simulink model "DP"  (Simulink 7.3)
settings: Solver=ode5  StartTime=0.0  StopTime=inf  FixedStep=0.1  RelTol=1e-3
undefined symbols (not defined in the file): eta1_0_real, v1_0_real, velocitySatValues1
libraries: simulink x18, marine_gnc x4, dspinverses x1, simulink_extras x1
(part 1 of 2)
settings Model: Creator=Dinh  LastModifiedBy=mcl  BufferReuse=off
settings DataIOCC: LimitDataPoints=off  SaveOutput=off  SaveTime=off
settings OptimizationCC: BlockReduction=off  BooleanDataType=off  ConditionallyExecuteInputs=off  OptimizeBlockIOStorage=off  BufferReuse=off  ExpressionFolding=off  LocalBlockOutputs=off  SimCompilerOptimization=On
settings SFSimCC: SimBuildMode=sf_nonincremental_build
settings RTWCC: SystemTargetFile=nidll_vxworks.tlc  TemplateMakefile=nidll_vxworks.tmf  Description=NI Real-Time VxWorks Target for Release 2007b or later  ProcessScript=nidll_vxworks_make_rtw_hook  RTWCompilerOptimization=On
settings STFCustomTargetCC: MatFileLogging=on  SystemTargetFile=nidll_vxworks.tlc

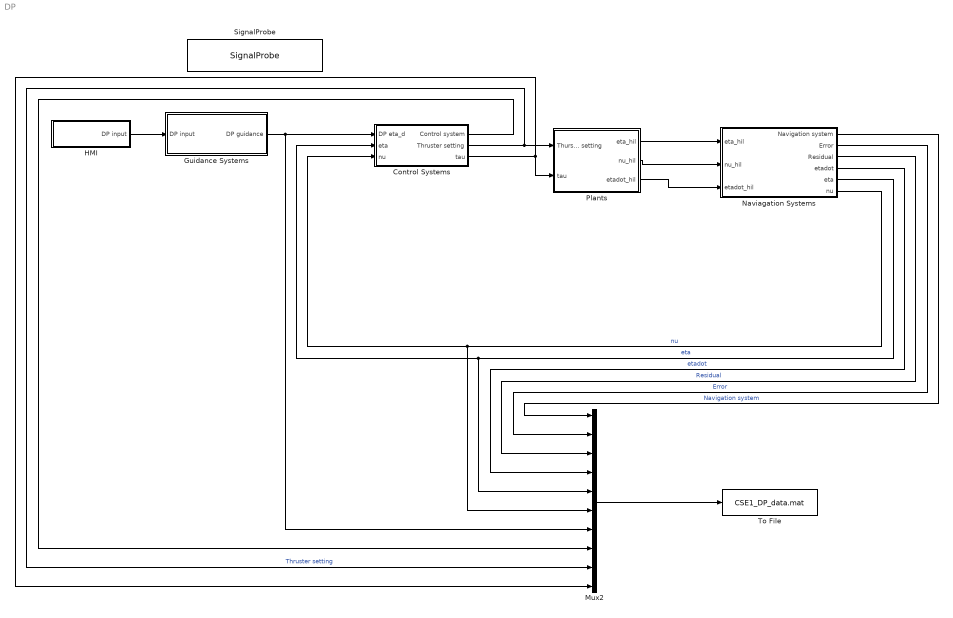
== system DP ==
  Control Systems : Subsystem
  Guidance Systems : Subsystem
  HMI : Subsystem
  Mux2 : Mux  Inputs=10
  Naviagation Systems : Subsystem
      settings: MinAlgLoopOccurrences=on
  Plants : Subsystem
  SignalProbe : S-Function  Description=Use this block with SIT.  FunctionName=SignalProbe  Parameters=1  EnableBusSupport=off
      settings: PreSaveFcn=NISIT_ModelVars;
      mask Description: The LabVIEW Simulation Interface Toolkit uses the SignalProbe block to probe the signals in the model. The SignalProbe block must be on the top level of the model hierarchy. You can have only one SignalProbe block per model file. Do not rename the SignalProbe block. Do not change the name of another model block to SignalProbe.
  To File : ToFile  Filename=CSE1_DP_data.mat  MatrixName=cse1_DP_data
  wires:
  HMI/1(DP input) -> Guidance Systems/1(DP input)
  Guidance Systems/1(DP guidance) -> Control Systems/1(DP eta_d), Mux2/7
  Plants/1(eta_hil) -> Naviagation Systems/1(eta_hil)
  Plants/2(nu_hil) -> Naviagation Systems/2(nu_hil)
  Plants/3(etadot_hil) -> Naviagation Systems/3(etadot_hil)
  Naviagation Systems/5(eta) -> Control Systems/2(eta), Mux2/5  "eta"
  Naviagation Systems/6(nu) -> Mux2/6, Control Systems/3(nu)  "nu"
  Naviagation Systems/3(Residual) -> Mux2/3  "Residual"
  Naviagation Systems/4(etadot) -> Mux2/4  "etadot"
  Naviagation Systems/2(Error) -> Mux2/2  "Error"
  Naviagation Systems/1(Navigation system) -> Mux2/1  "Navigation system"
  Mux2/1 -> To File/1
  Control Systems/1(Control system) -> Mux2/8
  Control Systems/3(tau) -> Mux2/10, Plants/2(tau)
  Control Systems/2(Thruster setting) -> Mux2/9, Plants/1(Thurster setting)  "Thruster setting"

== system DP/Control Systems ==
  note: 0 - PS3 u input control
      | 1 - DP control
  DP eta_d : Inport
  eta : Inport  Port=2
  nu : Inport  Port=3
  Control Mode : Constant  Value=0
  DP control : Subsystem
  PS3 input : Subsystem
  PS3 u input control : Subsystem
      settings: MinAlgLoopOccurrences=on
  Saturation : Saturate  UpperLimit=1.0  LowerLimit=-1.0
  Thruster setting Switch : MultiPortSwitch  Inputs=2  zeroidx=on
  tau Switch : MultiPortSwitch  Inputs=2  zeroidx=on
  Control system : Outport
  Thruster setting : Outport  Port=2
  tau : Outport  Port=3
  wires:
  Thruster setting Switch/1 -> Saturation/1
  Saturation/1 -> Thruster setting/1
  Control Mode/1 -> Thruster setting Switch/1, Control system/1, tau Switch/1
  PS3 u input control/1(Thruster setting) -> Thruster setting Switch/2
  PS3 input/1(DuelShock 3 signals) -> PS3 u input control/1(PS3 Signals)
  PS3 input/2(PS3 BT Power) -> PS3 u input control/2(PS3 BT Power)
  PS3 input/3(PS3 VSP Speed) -> PS3 u input control/3(PS3 VSP Speed)
  DP eta_d/1 -> DP control/1(eta_d)
  eta/1 -> DP control/2(eta)
  nu/1 -> DP control/3(nu)
  DP control/1(Thruster setting) -> Thruster setting Switch/3
  tau Switch/1 -> tau/1
  PS3 u input control/2(tau) -> tau Switch/2
  DP control/2(tau) -> tau Switch/3

== system DP/Guidance Systems ==
  DP input : Inport
  DP : Subsystem
  DP guidance : Outport
  wires:
  DP/1(DP eta_d) -> DP guidance/1
  DP input/1 -> DP/1(DP input)

== system DP/HMI ==
  Battery Bow Thruster : Gain  ParameterDataType=fixdt(1, 16)  ParameterScaling=2^0  OutDataType=fixdt(1, 16)  OutScaling=2^0
  Battery Main : Gain  Gain=2  ParameterDataType=fixdt(1, 16)  ParameterScaling=2^0  OutDataType=fixdt(1, 16)  OutScaling=2^0
  Battery Servo : Gain  ParameterDataType=fixdt(1, 16)  ParameterScaling=2^0  OutDataType=fixdt(1, 16)  OutScaling=2^0
  DP Input : Subsystem
  SIT zAI0 : S-Function  Priority=1  FunctionName=NI_SIT_IO  Parameters=width dtype portnum stime stype btype  EnableBusSupport=off  mask(SIT Inport){portnum=1, width=-1, stime=-1, dtype=auto, stype=auto, btype=1}
      mask prompts: portnum "Port number:"; width "Port dimensions (-1 for dynamically sized):"; stime "Sample time (-1 for inherited):"; dtype "Data type:"; stype "Signal type:"; btype "Block type:"
      mask help: Use this inport on any level of nested subsystems to allow the LabVIEW Simulation Interface Toolkit to map hardware to it.
      mask init:
      | NI_SIT_IO_init;
      settings: CopyFcn=NI_SIT_IO_callbacks(1);  DeleteFcn=NI_SIT_IO_callbacks(2);
      mask StyleString: edit,edit,edit,popup(auto|double|single|int8|uint8|int16|uint16|int32|uint32|boolean),popup(auto|real|complex),edit
      mask CallbackString: NI_SIT_IO_callbacks(3);|||NI_SIT_IO_callbacks(4);||
      mask TabNameString: Parameters,Parameters,Parameters,Parameters,Parameters,Parameters
      mask Display:
      | patch([-x x], [-y y], [.90980 .81960 .32156]);
      | plot([0 -x x 0], [rad -y y rad]);
      | fprintf('SIT%d', portnum);
  SIT zAI1 : S-Function  Priority=2  FunctionName=NI_SIT_IO  Parameters=width dtype portnum stime stype btype  EnableBusSupport=off  mask(SIT Inport){portnum=2, width=-1, stime=-1, dtype=auto, stype=auto, btype=1}
      mask prompts: portnum "Port number:"; width "Port dimensions (-1 for dynamically sized):"; stime "Sample time (-1 for inherited):"; dtype "Data type:"; stype "Signal type:"; btype "Block type:"
      mask help: Use this inport on any level of nested subsystems to allow the LabVIEW Simulation Interface Toolkit to map hardware to it.
      mask init:
      | NI_SIT_IO_init;
      settings: CopyFcn=NI_SIT_IO_callbacks(1);  DeleteFcn=NI_SIT_IO_callbacks(2);
      mask StyleString: edit,edit,edit,popup(auto|double|single|int8|uint8|int16|uint16|int32|uint32|boolean),popup(auto|real|complex),edit
      mask CallbackString: NI_SIT_IO_callbacks(3);|||NI_SIT_IO_callbacks(4);||
      mask TabNameString: Parameters,Parameters,Parameters,Parameters,Parameters,Parameters
      mask Display:
      | patch([-x x], [-y y], [.90980 .81960 .32156]);
      | plot([0 -x x 0], [rad -y y rad]);
      | fprintf('SIT%d', portnum);
  SIT zAI2 : S-Function  Priority=3  FunctionName=NI_SIT_IO  Parameters=width dtype portnum stime stype btype  EnableBusSupport=off  mask(SIT Inport){portnum=3, width=-1, stime=-1, dtype=auto, stype=auto, btype=1}
      mask prompts: portnum "Port number:"; width "Port dimensions (-1 for dynamically sized):"; stime "Sample time (-1 for inherited):"; dtype "Data type:"; stype "Signal type:"; btype "Block type:"
      mask help: Use this inport on any level of nested subsystems to allow the LabVIEW Simulation Interface Toolkit to map hardware to it.
      mask init:
      | NI_SIT_IO_init;
      settings: CopyFcn=NI_SIT_IO_callbacks(1);  DeleteFcn=NI_SIT_IO_callbacks(2);
      mask StyleString: edit,edit,edit,popup(auto|double|single|int8|uint8|int16|uint16|int32|uint32|boolean),popup(auto|real|complex),edit
      mask CallbackString: NI_SIT_IO_callbacks(3);|||NI_SIT_IO_callbacks(4);||
      mask TabNameString: Parameters,Parameters,Parameters,Parameters,Parameters,Parameters
      mask Display:
      | patch([-x x], [-y y], [.90980 .81960 .32156]);
      | plot([0 -x x 0], [rad -y y rad]);
      | fprintf('SIT%d', portnum);
  Terminator Bow Thruster Battery : Terminator
  Terminator Main Battery : Terminator
  Terminator Servo Battery : Terminator
  DP input : Outport
  wires:
  SIT zAI0/1 -> Battery Bow Thruster/1
  SIT zAI1/1 -> Battery Servo/1
  SIT zAI2/1 -> Battery Main/1
  Battery Bow Thruster/1 -> Terminator Bow Thruster Battery/1
  Battery Servo/1 -> Terminator Servo Battery/1
  Battery Main/1 -> Terminator Main Battery/1
  DP Input/1(DP input) -> DP input/1

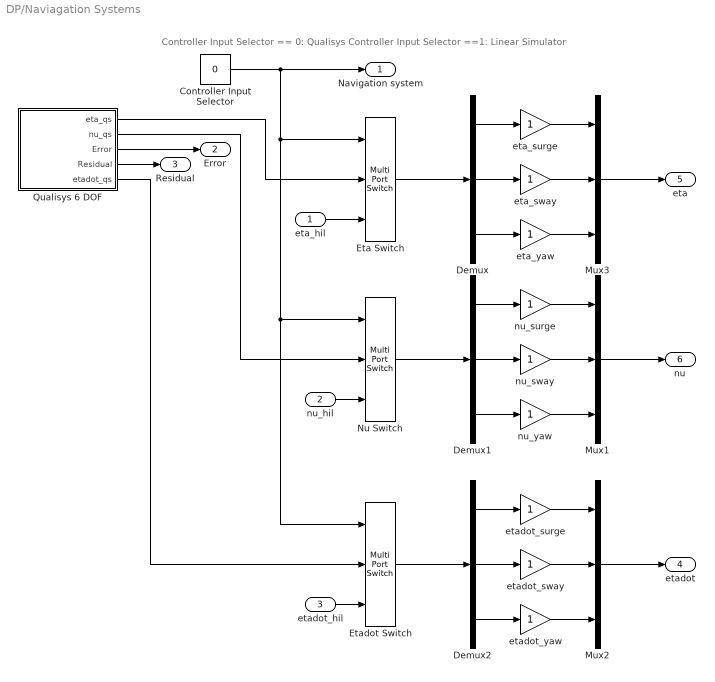
== system DP/Naviagation Systems ==
  note: Controller Input Selector == 0: Qualisys
      | Controller Input Selector ==1: Linear Simulator
  eta_hil : Inport
  nu_hil : Inport  Port=2
  etadot_hil : Inport  Port=3
  Controller Input Selector : Constant  Value=0
  Demux : Demux  Outputs=3
  Demux1 : Demux  Outputs=3
  Demux2 : Demux  Outputs=3
  Eta Switch : MultiPortSwitch  Inputs=2  zeroidx=on
  Etadot Switch : MultiPortSwitch  Inputs=2  zeroidx=on
  Mux1 : Mux  Inputs=3
  Mux2 : Mux  Inputs=3
  Mux3 : Mux  Inputs=3
  Nu Switch : MultiPortSwitch  Inputs=2  zeroidx=on
  Qualisys 6 DOF : Subsystem
  eta_surge : Gain  ParameterDataType=fixdt(1, 16)  ParameterScaling=2^0  OutDataType=fixdt(1, 16)  OutScaling=2^0
  eta_sway : Gain  ParameterDataType=fixdt(1, 16)  ParameterScaling=2^0  OutDataType=fixdt(1, 16)  OutScaling=2^0
  eta_yaw : Gain  ParameterDataType=fixdt(1, 16)  ParameterScaling=2^0  OutDataType=fixdt(1, 16)  OutScaling=2^0
  etadot_surge : Gain  ParameterDataType=fixdt(1, 16)  ParameterScaling=2^0  OutDataType=fixdt(1, 16)  OutScaling=2^0
  etadot_sway : Gain  ParameterDataType=fixdt(1, 16)  ParameterScaling=2^0  OutDataType=fixdt(1, 16)  OutScaling=2^0
  etadot_yaw : Gain  ParameterDataType=fixdt(1, 16)  ParameterScaling=2^0  OutDataType=fixdt(1, 16)  OutScaling=2^0
  nu_surge : Gain  ParameterDataType=fixdt(1, 16)  ParameterScaling=2^0  OutDataType=fixdt(1, 16)  OutScaling=2^0
  nu_sway : Gain  ParameterDataType=fixdt(1, 16)  ParameterScaling=2^0  OutDataType=fixdt(1, 16)  OutScaling=2^0
  nu_yaw : Gain  ParameterDataType=fixdt(1, 16)  ParameterScaling=2^0  OutDataType=fixdt(1, 16)  OutScaling=2^0
  Navigation system : Outport
  Error : Outport  Port=2
  Residual : Outport  Port=3
  etadot : Outport  Port=4
  eta : Outport  Port=5
  nu : Outport  Port=6
  wires:
  Controller Input Selector/1 -> Eta Switch/1, Nu Switch/1, Etadot Switch/1, Navigation system/1
  Qualisys 6 DOF/1(eta_qs) -> Eta Switch/2
  Qualisys 6 DOF/2(nu_qs) -> Nu Switch/2
  eta_hil/1 -> Eta Switch/3
  nu_hil/1 -> Nu Switch/3
  Demux/1 -> eta_surge/1
  Demux/2 -> eta_sway/1
  Demux/3 -> eta_yaw/1
  eta_surge/1 -> Mux3/1
  eta_yaw/1 -> Mux3/3
  eta_sway/1 -> Mux3/2
  Mux3/1 -> eta/1
  Demux1/1 -> nu_surge/1
  Demux1/2 -> nu_sway/1
  Demux1/3 -> nu_yaw/1
  nu_surge/1 -> Mux1/1
  nu_sway/1 -> Mux1/2
  nu_yaw/1 -> Mux1/3
  Mux1/1 -> nu/1
  Nu Switch/1 -> Demux1/1
  Eta Switch/1 -> Demux/1
  Qualisys 6 DOF/3(Error) -> Error/1
  Qualisys 6 DOF/4(Residual) -> Residual/1
  Demux2/1 -> etadot_surge/1
  Demux2/2 -> etadot_sway/1
  Demux2/3 -> etadot_yaw/1
  etadot_surge/1 -> Mux2/1
  etadot_yaw/1 -> Mux2/3
  etadot_sway/1 -> Mux2/2
  Mux2/1 -> etadot/1
  Etadot Switch/1 -> Demux2/1
  Qualisys 6 DOF/5(etadot_qs) -> Etadot Switch/2
  etadot_hil/1 -> Etadot Switch/3

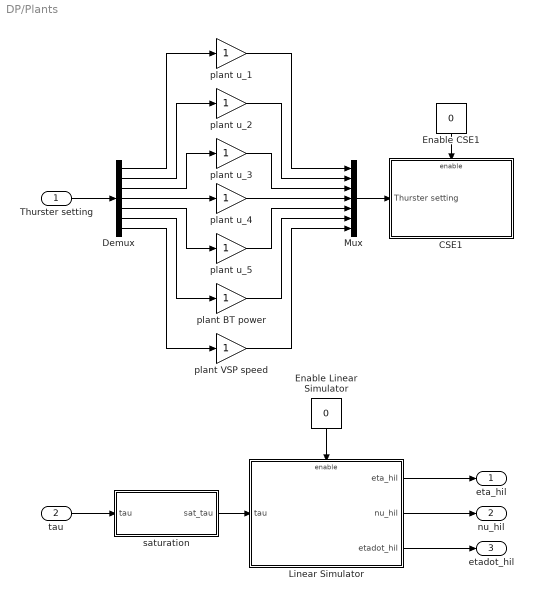
== system DP/Plants ==
  Thurster setting : Inport
  tau : Inport  Port=2
  CSE1 : Subsystem
  Demux : Demux  Outputs=7
  Enable CSE1 : Constant  Value=0
  Enable Linear Simulator : Constant  Value=0
  Linear Simulator : Subsystem
      settings: MinAlgLoopOccurrences=on
  Mux : Mux  Inputs=7
  plant BT power : Gain  ParameterDataType=fixdt(1, 16)  ParameterScaling=2^0  OutDataType=fixdt(1, 16)  OutScaling=2^0
  plant VSP speed : Gain  ParameterDataType=fixdt(1, 16)  ParameterScaling=2^0  OutDataType=fixdt(1, 16)  OutScaling=2^0
  plant u_{1..5} (5 alike) : Gain  ParameterDataType=fixdt(1, 16)  ParameterScaling=2^0  OutDataType=fixdt(1, 16)  OutScaling=2^0
  saturation : Subsystem
  eta_hil : Outport
  nu_hil : Outport  Port=2
  etadot_hil : Outport  Port=3
  wires:
  Enable CSE1/1 -> CSE1/Enable
  Thurster setting/1 -> Demux/1
  Mux/1 -> CSE1/1(Thurster setting)
  Demux/1 -> plant u_1/1
  Demux/2 -> plant u_2/1
  Demux/3 -> plant u_3/1
  Demux/4 -> plant u_4/1
  plant u_4/1 -> Mux/4
  plant u_1/1 -> Mux/1
  plant u_2/1 -> Mux/2
  plant u_3/1 -> Mux/3
  Demux/5 -> plant u_5/1
  Demux/6 -> plant BT power/1
  Demux/7 -> plant VSP speed/1
  plant u_5/1 -> Mux/5
  plant BT power/1 -> Mux/6
  plant VSP speed/1 -> Mux/7
  Linear Simulator/1(eta_hil) -> eta_hil/1
  Linear Simulator/2(nu_hil) -> nu_hil/1
  Enable Linear Simulator/1 -> Linear Simulator/Enable
  tau/1 -> saturation/1(tau)
  saturation/1(sat_tau) -> Linear Simulator/1(tau)
  Linear Simulator/3(etadot_hil) -> etadot_hil/1

== system DP/Control Systems/DP control ==
  note: This subsystem is a modifired version of Håkon Skåtuns subsystem of same name
  eta_d : Inport
  eta : Inport  Port=2
  nu : Inport  Port=3
  BT_power_limit : Constant  Value=0.5
  DP controller : Subsystem  mask(Nonlinear DP Controller){Kp=(0.1)^2*[25.8000 0  0;  0  33.8000  1.0115;  0  1.0115  2.7600 ], Kd=2*0.8*0.1*[25.8000 0  0;  0  33.8000  1.0115;  0  1.0115  2.7600 ], Ki=(0.1^3/10)*[25.8000 0  0;  0  33.8000  1.0115;  0  1.0115  2.7600 ]}
      mask prompts: Kp "Proportional Gain Matrix: Kp"; Kd "Derivative Gain Matrix: Kd"; Ki "Integral Gain Matrix: Ki"
      mask help: Nonlinear PID controller for Set-Point Reulation in Surge, Sway and Yaw
      mask Help:
      | The nonlinear  PID controller uses the rotation matrix in yaw for proper scaling of the surge, sway and yaw gains as a function of the yaw angle.
      | INPUTS: (1) eta_ref, (2) eta, (3) nu. OUPUTS: (1) tau.
      mask Display: disp('Nonlinear PID\n set-point controller')
  Mux1 : Mux  Inputs=3
  Saturation : Saturate  UpperLimit=1.0  LowerLimit=-1.0
  Thruster allocation : Subsystem
  VSP_speeds : Constant  Value=0.4
  Thruster setting : Outport  InitialOutput=[0;0;0;0;0;0;0]
  tau : Outport  Port=2
  wires:
  Mux1/1 -> Thruster setting/1
  eta_d/1 -> DP controller/1(eta_ref)
  eta/1 -> DP controller/2(eta)
  nu/1 -> DP controller/3(nu)
  Saturation/1 -> Mux1/1
  BT_power_limit/1 -> Mux1/2
  VSP_speeds/1 -> Mux1/3
  Thruster allocation/1(u_act) -> Saturation/1
  DP controller/1(tau) -> Thruster allocation/1(tau), tau/1

== system DP/Control Systems/PS3 input ==
  note: Y-axis of analog sticks points up (in the direction of the shoulder buttons),
      | while  X-axis points to the right (in the direction of
      | Triange, Circle, X and Square buttons)
  AS_LX : Constant  Value=0
  AS_LY : Constant  Value=0
  AS_RX : Constant  Value=0
  AS_RY : Constant  Value=0
  L2 : Constant  Value=0
  Mux : Mux  Inputs=6
  PS3_BT_Power : Constant  Value=0
  PS3_VSP_Speed : Constant  Value=0
  R2 : Constant  Value=0
  ScalingLX : Gain  Gain=1/32767
  ScalingLY : Gain  Gain=1/32767
  ScalingRY : Gain  Gain=1/32767
  Scaling_RX : Gain  Gain=1/32767
  DuelShock 3 signals : Outport
  PS3 BT Power : Outport  Port=2
  PS3 VSP Speed : Outport  Port=3
  wires:
  PS3_VSP_Speed/1 -> PS3 VSP Speed/1  "Voith Schnider Propeller Speed"
  PS3_BT_Power/1 -> PS3 BT Power/1  "Bow Thruster Power limit"
  Mux/1 -> DuelShock 3 signals/1
  AS_LX/1 -> ScalingLX/1  "x-position of left analog stick [-32767,32767]"
  ScalingLX/1 -> Mux/1  "x-position of left analog stick [-1,1]"
  AS_LY/1 -> ScalingLY/1  "y-position of left analog stick [-32767,32767]"
  ScalingLY/1 -> Mux/2  "y-position of left analog stick [-1,1]"
  AS_RX/1 -> Scaling_RX/1  "x-position of right analog stick  [-32767,32767]"
  Scaling_RX/1 -> Mux/3  "x-position of right analog stick  [-1,1]"
  ScalingRY/1 -> Mux/4  "y-position of right analog stick [-1,1]"
  AS_RY/1 -> ScalingRY/1  "y-position of right analog stick [-32767,32767]"
  L2/1 -> Mux/5  "L2 Button [-1,0]"
  R2/1 -> Mux/6  "R2 Button [0,1]"

== system DP/Control Systems/PS3 u input control ==
  note: Manuel thruster control is intended for testing and flexing of thrusters and its signals
  note: Mapping PS3 signals to thruster settings:
      | - Y-position controls surge force of VSP
      | - X-positon controls sway force of VSP
      | - Left Analogstick controls port VSP
      | - Right Analogstick controls starboard VSP
      | - Postive values gives postive motions and vice versa
      | - R2 pressed gives postive yaw motion
      | - L2 pressed gives negative yaw motion
  PS3 Signals : Inport
  PS3 BT Power : Inport  Port=2
  PS3 VSP Speed : Inport  Port=3
  Add : Sum  Inputs=|++
  Demux : Demux  Outputs=6
  Mux : Mux  Inputs=7
  PS3 u_{1..5} (5 alike) : Gain  ParameterDataType=fixdt(1, 16)  ParameterScaling=2^0  OutDataType=fixdt(1, 16)  OutScaling=2^0
  Subsystem : Subsystem
  Thruster setting : Outport
  tau : Outport  Port=2
  wires:
  PS3 Signals/1 -> Demux/1
  Demux/1 -> PS3 u_2/1  "Left/Right position of Left Analogstick"
  Demux/2 -> PS3 u_1/1  "Up/Down position of Left Analogstick"
  Demux/3 -> PS3 u_4/1  "Left/Right position of Right Analogstick"
  Demux/4 -> PS3 u_3/1  "Up/Down position of Right Analogstick"
  Demux/5 -> Add/1  "L2 signal"
  Demux/6 -> Add/2  "R2 signal"
  PS3 VSP Speed/1 -> Mux/7  "VPS Speed"
  PS3 BT Power/1 -> Mux/6  "Bow Thruster Limit"
  Add/1 -> PS3 u_5/1  "Bow Thruster direction"
  Mux/1 -> Thruster setting/1, Subsystem/1(u_act)
  PS3 u_1/1 -> Mux/1  "u_1"
  PS3 u_2/1 -> Mux/2  "u_2"
  PS3 u_5/1 -> Mux/5  "u_5"
  PS3 u_4/1 -> Mux/4  "u_4"
  PS3 u_3/1 -> Mux/3  "u_3"
  Subsystem/1(tau) -> tau/1

== system DP/Guidance Systems/DP ==
  DP input : Inport
  Demux1 : Demux  Outputs=3
  Mux : Mux  Inputs=3
  eta_d DP E : Gain  ParameterDataType=fixdt(1, 16)  ParameterScaling=2^0  OutDataType=fixdt(1, 16)  OutScaling=2^0
  eta_d DP N : Gain  ParameterDataType=fixdt(1, 16)  ParameterScaling=2^0  OutDataType=fixdt(1, 16)  OutScaling=2^0
  eta_d DP Psi : Gain  ParameterDataType=fixdt(1, 16)  ParameterScaling=2^0  OutDataType=fixdt(1, 16)  OutScaling=2^0
  DP eta_d : Outport
  wires:
  DP input/1 -> Demux1/1
  eta_d DP N/1 -> Mux/1
  eta_d DP E/1 -> Mux/2
  eta_d DP Psi/1 -> Mux/3
  Demux1/1 -> eta_d DP N/1
  Demux1/2 -> eta_d DP E/1
  Demux1/3 -> eta_d DP Psi/1
  Mux/1 -> DP eta_d/1

== system DP/HMI/DP Input ==
  Degrees to Radians : simulink_extras/Transformations/Degrees to Radians  SystemSampleTime=-1
  Mux : Mux  Inputs=3
  psi_d : Constant  Value=0
  x_d : Constant  Value=0
  y_d : Constant  Value=0
  DP input : Outport
  wires:
  x_d/1 -> Mux/1
  y_d/1 -> Mux/2
  Mux/1 -> DP input/1
  psi_d/1 -> Degrees to Radians/1
  Degrees to Radians/1 -> Mux/3

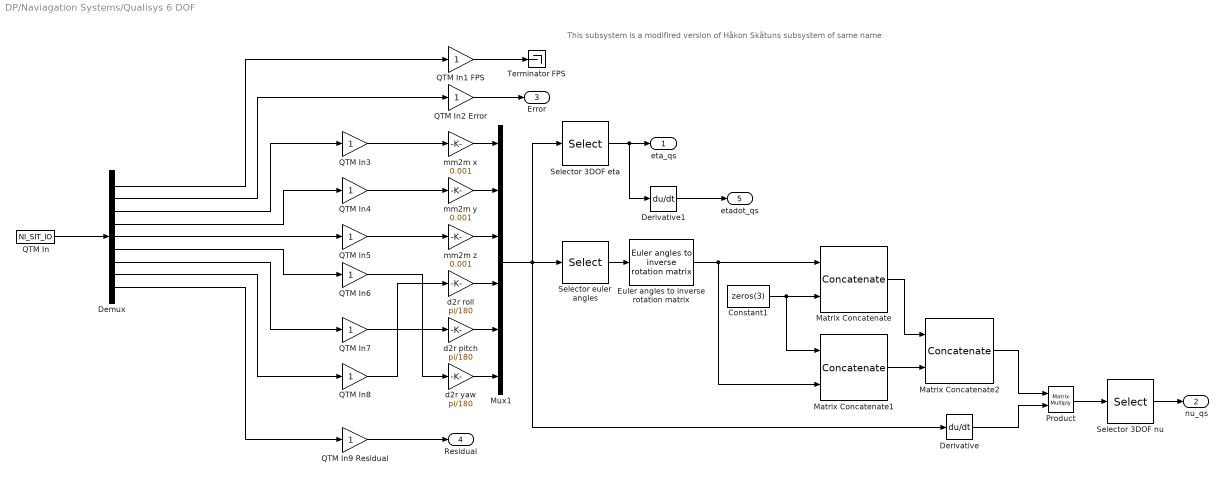
== system DP/Naviagation Systems/Qualisys 6 DOF ==
  note: This subsystem is a modifired version of Håkon Skåtuns subsystem of same name
  Constant1 : Constant  Value=zeros(3)
  Demux : Demux  Outputs=9
  Derivative : Derivative
  Derivative1 : Derivative
  Euler angles to inverse rotation matrix : marine_gnc/Models/ Kinematics/Euler angles to inverse rotation matrix  SystemSampleTime=-1
  Matrix Concatenate : Concatenate  Mode=Multidimensional array
  Matrix Concatenate1 : Concatenate  Mode=Multidimensional array
  Matrix Concatenate2 : Concatenate  Mode=Multidimensional array  ConcatenateDimension=2
  Mux1 : Mux  Inputs=6
  Product : Product  Multiplication=Matrix(*)  RndMeth=Zero
  QTM In : S-Function  Priority=1  FunctionName=NI_SIT_IO  Parameters=width dtype portnum stime stype btype  EnableBusSupport=off  mask(SIT Inport){portnum=1, width=9, stime=-1, dtype=auto, stype=auto, btype=1}
      mask prompts: portnum "Port number:"; width "Port dimensions (-1 for dynamically sized):"; stime "Sample time (-1 for inherited):"; dtype "Data type:"; stype "Signal type:"; btype "Block type:"
      mask help: Use this inport on any level of nested subsystems to allow the LabVIEW Simulation Interface Toolkit to map hardware to it.
      mask init:
      | NI_SIT_IO_init;
      settings: CopyFcn=NI_SIT_IO_callbacks(1);  DeleteFcn=NI_SIT_IO_callbacks(2);
      mask StyleString: edit,edit,edit,popup(auto|double|single|int8|uint8|int16|uint16|int32|uint32|boolean),popup(auto|real|complex),edit
      mask CallbackString: NI_SIT_IO_callbacks(3);|||NI_SIT_IO_callbacks(4);||
      mask TabNameString: Parameters,Parameters,Parameters,Parameters,Parameters,Parameters
      mask Display:
      | patch([-x x], [-y y], [.90980 .81960 .32156]);
      | plot([0 -x x 0], [rad -y y rad]);
      | fprintf('SIT%d', portnum);
  QTM In1 FPS : Gain  ParameterDataType=fixdt(1, 16)  ParameterScaling=2^0  OutDataType=fixdt(1, 16)  OutScaling=2^0
  QTM In2 Error : Gain  ParameterDataType=fixdt(1, 16)  ParameterScaling=2^0  OutDataType=fixdt(1, 16)  OutScaling=2^0
  QTM In{3..8} (6 alike) : Gain  ParameterDataType=fixdt(1, 16)  ParameterScaling=2^0  OutDataType=fixdt(1, 16)  OutScaling=2^0
  QTM In9 Residual : Gain  ParameterDataType=fixdt(1, 16)  ParameterScaling=2^0  OutDataType=fixdt(1, 16)  OutScaling=2^0
  Selector 3DOF eta : Selector  InputPortWidth=6  IndexOptions=Index vector (dialog)  Indices=[1 2 6]  OutputSizes=1
  Selector 3DOF nu : Selector  InputPortWidth=6  IndexOptions=Index vector (dialog)  Indices=[1 2 6]  OutputSizes=1
  Selector euler angles : Selector  InputPortWidth=6  IndexOptions=Index vector (dialog)  Indices=[4 5 6]  OutputSizes=1
  Terminator FPS : Terminator
  d2r pitch : Gain  Gain=pi/180  ParameterDataType=fixdt(1, 16)  ParameterScaling=2^0  OutDataType=fixdt(1, 16)  OutScaling=2^0
  d2r roll : Gain  Gain=pi/180  ParameterDataType=fixdt(1, 16)  ParameterScaling=2^0  OutDataType=fixdt(1, 16)  OutScaling=2^0
  d2r yaw : Gain  Gain=pi/180  ParameterDataType=fixdt(1, 16)  ParameterScaling=2^0  OutDataType=fixdt(1, 16)  OutScaling=2^0
  mm2m x : Gain  Gain=0.001
  mm2m y : Gain  Gain=0.001
  mm2m z : Gain  Gain=0.001
  eta_qs : Outport
  nu_qs : Outport  Port=2
  Error : Outport  Port=3
  Residual : Outport  Port=4
  etadot_qs : Outport  Port=5
  wires:
  Mux1/1 -> Selector euler angles/1, Derivative/1, Selector 3DOF eta/1
  Selector 3DOF eta/1 -> eta_qs/1, Derivative1/1
  Euler angles to inverse rotation matrix/1 -> Matrix Concatenate/1, Matrix Concatenate1/2
  Matrix Concatenate/1 -> Matrix Concatenate2/1
  Matrix Concatenate1/1 -> Matrix Concatenate2/2
  Matrix Concatenate2/1 -> Product/1
  Derivative/1 -> Product/2
  Constant1/1 -> Matrix Concatenate/2, Matrix Concatenate1/1
  mm2m z/1 -> Mux1/3
  mm2m y/1 -> Mux1/2
  mm2m x/1 -> Mux1/1
  d2r yaw/1 -> Mux1/6
  d2r pitch/1 -> Mux1/5
  d2r roll/1 -> Mux1/4
  Selector euler angles/1 -> Euler angles to inverse rotation matrix/1
  Product/1 -> Selector 3DOF nu/1
  Selector 3DOF nu/1 -> nu_qs/1
  QTM In1 FPS/1 -> Terminator FPS/1
  QTM In2 Error/1 -> Error/1
  QTM In9 Residual/1 -> Residual/1
  QTM In/1 -> Demux/1
  Demux/1 -> QTM In1 FPS/1
  Demux/2 -> QTM In2 Error/1
  Demux/3 -> QTM In3/1
  Demux/4 -> QTM In4/1
  Demux/5 -> QTM In5/1
  Demux/6 -> QTM In6/1
  Demux/7 -> QTM In7/1
  Demux/8 -> QTM In8/1
  Demux/9 -> QTM In9 Residual/1
  QTM In3/1 -> mm2m x/1
  QTM In4/1 -> mm2m y/1
  QTM In5/1 -> mm2m z/1
  QTM In7/1 -> d2r pitch/1
  QTM In6/1 -> d2r yaw/1
  QTM In8/1 -> d2r roll/1
  Derivative1/1 -> etadot_qs/1

== system DP/Plants/CSE1 ==
  note: This subsystem is a modifired version of Håkon Skåtuns subsystem CSE1
  Thurster setting : Inport
  Enable : EnablePort  StatesWhenEnabling=reset
  Bow Thruster : Subsystem
  Demux : Demux  Outputs=7
  "Voith Schneider Propeller " : Subsystem
  wires:
  Thurster setting/1 -> Demux/1
  Demux/1 -> "Voith Schneider Propeller "/1(Port VSP y u_1)
  Demux/2 -> "Voith Schneider Propeller "/2(Port VSP x u_2)
  Demux/3 -> "Voith Schneider Propeller "/3(Starboard VSP y u_3)
  Demux/4 -> "Voith Schneider Propeller "/4(Starboard VSP x u_4)
  Demux/7 -> "Voith Schneider Propeller "/5(VSP Speed)
  Demux/5 -> Bow Thruster/1(Bow Thruster Direction u_5)
  Demux/6 -> Bow Thruster/2(Bow Thruster Power)

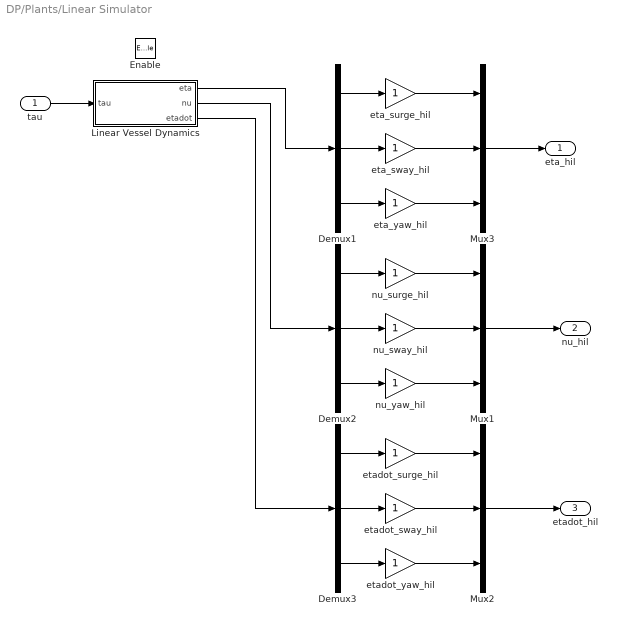
== system DP/Plants/Linear Simulator ==
  tau : Inport
  Enable : EnablePort  StatesWhenEnabling=reset
  Demux1 : Demux  Outputs=3
  Demux2 : Demux  Outputs=3
  Demux3 : Demux  Outputs=3
  Linear Vessel Dynamics : Subsystem
  Mux1 : Mux  Inputs=3
  Mux2 : Mux  Inputs=3
  Mux3 : Mux  Inputs=3
  eta_surge_hil : Gain  ParameterDataType=fixdt(1, 16)  ParameterScaling=2^0  OutDataType=fixdt(1, 16)  OutScaling=2^0
  eta_sway_hil : Gain  ParameterDataType=fixdt(1, 16)  ParameterScaling=2^0  OutDataType=fixdt(1, 16)  OutScaling=2^0
  eta_yaw_hil : Gain  ParameterDataType=fixdt(1, 16)  ParameterScaling=2^0  OutDataType=fixdt(1, 16)  OutScaling=2^0
  etadot_surge_hil : Gain  ParameterDataType=fixdt(1, 16)  ParameterScaling=2^0  OutDataType=fixdt(1, 16)  OutScaling=2^0
  etadot_sway_hil : Gain  ParameterDataType=fixdt(1, 16)  ParameterScaling=2^0  OutDataType=fixdt(1, 16)  OutScaling=2^0
  etadot_yaw_hil : Gain  ParameterDataType=fixdt(1, 16)  ParameterScaling=2^0  OutDataType=fixdt(1, 16)  OutScaling=2^0
  nu_surge_hil : Gain  ParameterDataType=fixdt(1, 16)  ParameterScaling=2^0  OutDataType=fixdt(1, 16)  OutScaling=2^0
  nu_sway_hil : Gain  ParameterDataType=fixdt(1, 16)  ParameterScaling=2^0  OutDataType=fixdt(1, 16)  OutScaling=2^0
  nu_yaw_hil : Gain  ParameterDataType=fixdt(1, 16)  ParameterScaling=2^0  OutDataType=fixdt(1, 16)  OutScaling=2^0
  eta_hil : Outport
  nu_hil : Outport  Port=2
  etadot_hil : Outport  Port=3
  wires:
  nu_yaw_hil/1 -> Mux1/3
  nu_sway_hil/1 -> Mux1/2
  nu_surge_hil/1 -> Mux1/1
  Demux2/3 -> nu_yaw_hil/1
  Demux2/2 -> nu_sway_hil/1
  Demux2/1 -> nu_surge_hil/1
  eta_sway_hil/1 -> Mux3/2
  eta_yaw_hil/1 -> Mux3/3
  eta_surge_hil/1 -> Mux3/1
  Demux1/3 -> eta_yaw_hil/1
  Demux1/2 -> eta_sway_hil/1
  Demux1/1 -> eta_surge_hil/1
  Linear Vessel Dynamics/1(eta) -> Demux1/1
  Linear Vessel Dynamics/2(nu) -> Demux2/1
  Mux1/1 -> nu_hil/1
  Mux3/1 -> eta_hil/1
  etadot_sway_hil/1 -> Mux2/2
  etadot_yaw_hil/1 -> Mux2/3
  etadot_surge_hil/1 -> Mux2/1
  Demux3/3 -> etadot_yaw_hil/1
  Demux3/2 -> etadot_sway_hil/1
  Demux3/1 -> etadot_surge_hil/1
  Linear Vessel Dynamics/3(etadot) -> Demux3/1
  Mux2/1 -> etadot_hil/1
  tau/1 -> Linear Vessel Dynamics/1(tau)

== system DP/Plants/saturation ==
  tau : Inport  OutDataType=sfix(16)  OutScaling=2^0
  Demux : Demux  Outputs=3
  Mux1 : Mux  Inputs=3
  Saturation : Saturate  UpperLimit=3  LowerLimit=-2.6  OutDataType=fixdt(1, 16)  OutScaling=2^0
  Saturation1 : Saturate  UpperLimit=3  LowerLimit=-3.5  OutDataType=fixdt(1, 16)  OutScaling=2^0
  Saturation2 : Saturate  UpperLimit=1.6  LowerLimit=-1.5  OutDataType=fixdt(1, 16)  OutScaling=2^0
  plant tau_surge : Gain  ParameterDataType=fixdt(1, 16)  ParameterScaling=2^0  OutDataType=fixdt(1, 16)  OutScaling=2^0
  plant tau_sway : Gain  ParameterDataType=fixdt(1, 16)  ParameterScaling=2^0  OutDataType=fixdt(1, 16)  OutScaling=2^0
  plant tau_yaw : Gain  ParameterDataType=fixdt(1, 16)  ParameterScaling=2^0  OutDataType=fixdt(1, 16)  OutScaling=2^0
  sat_tau : Outport  OutDataType=sfix(16)  OutScaling=2^0
  wires:
  Mux1/1 -> sat_tau/1
  tau/1 -> Demux/1
  Saturation/1 -> plant tau_surge/1
  Demux/1 -> Saturation/1
  Demux/2 -> Saturation1/1
  Saturation1/1 -> plant tau_sway/1
  plant tau_surge/1 -> Mux1/1
  plant tau_sway/1 -> Mux1/2
  Demux/3 -> Saturation2/1
  Saturation2/1 -> plant tau_yaw/1
  plant tau_yaw/1 -> Mux1/3

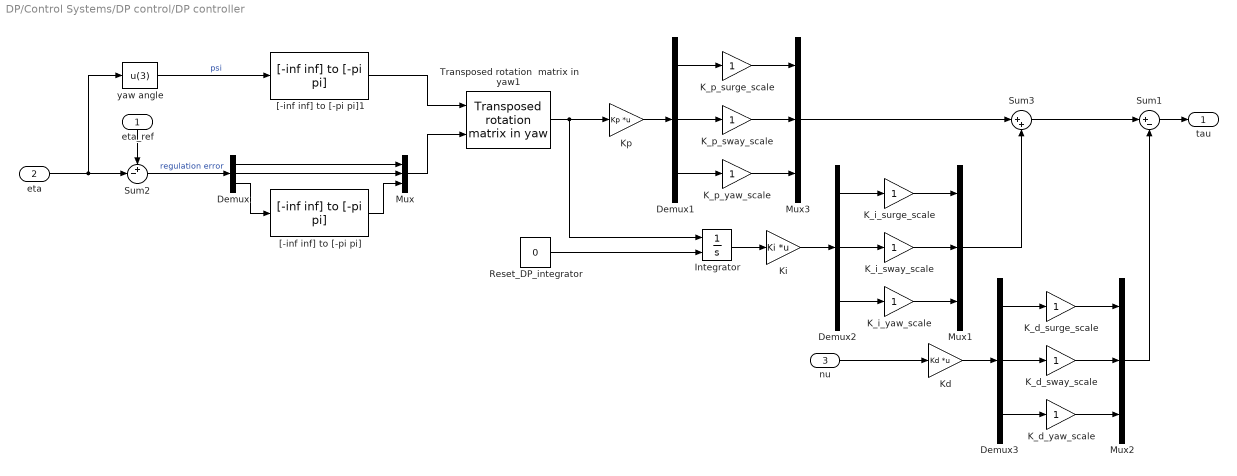
== system DP/Control Systems/DP control/DP controller ==
  eta_ref : Inport
  eta : Inport  Port=2
  nu : Inport  Port=3
  Demux{,1..3} (4 alike) : Demux  Outputs=3
  Integrator : Integrator  ExternalReset=level
  K_d_surge_scale : Gain  ParameterDataType=fixdt(1, 16)  ParameterScaling=2^0  OutDataType=fixdt(1, 16)  OutScaling=2^0
  K_d_sway_scale : Gain  ParameterDataType=fixdt(1, 16)  ParameterScaling=2^0  OutDataType=fixdt(1, 16)  OutScaling=2^0
  K_d_yaw_scale : Gain  ParameterDataType=fixdt(1, 16)  ParameterScaling=2^0  OutDataType=fixdt(1, 16)  OutScaling=2^0
  K_i_surge_scale : Gain  ParameterDataType=fixdt(1, 16)  ParameterScaling=2^0  OutDataType=fixdt(1, 16)  OutScaling=2^0
  K_i_sway_scale : Gain  ParameterDataType=fixdt(1, 16)  ParameterScaling=2^0  OutDataType=fixdt(1, 16)  OutScaling=2^0
  K_i_yaw_scale : Gain  ParameterDataType=fixdt(1, 16)  ParameterScaling=2^0  OutDataType=fixdt(1, 16)  OutScaling=2^0
  K_p_surge_scale : Gain  ParameterDataType=fixdt(1, 16)  ParameterScaling=2^0  OutDataType=fixdt(1, 16)  OutScaling=2^0
  K_p_sway_scale : Gain  ParameterDataType=fixdt(1, 16)  ParameterScaling=2^0  OutDataType=fixdt(1, 16)  OutScaling=2^0
  K_p_yaw_scale : Gain  ParameterDataType=fixdt(1, 16)  ParameterScaling=2^0  OutDataType=fixdt(1, 16)  OutScaling=2^0
  Kd : Gain  Gain=Kd  Multiplication=Matrix(K*u)  SaturateOnIntegerOverflow=on  OutDataTypeStr=Inherit: Same as input  ParamDataTypeStr=Inherit: Same as input
  Ki : Gain  Gain=Ki  Multiplication=Matrix(K*u)  SaturateOnIntegerOverflow=on  OutDataTypeStr=Inherit: Same as input  ParamDataTypeStr=Inherit: Same as input
  Kp : Gain  Gain=Kp  Multiplication=Matrix(K*u)  SaturateOnIntegerOverflow=on  OutDataTypeStr=Inherit: Same as input  ParamDataTypeStr=Inherit: Same as input
  Mux{,1..3} (4 alike) : Mux  Inputs=3
  Reset_DP_integrator : Constant  Value=0
  Sum1 : Sum  Inputs=|+-  SaturateOnIntegerOverflow=on  InputSameDT=on  OutDataTypeStr=Inherit: Same as first input
  Sum2 : Sum  Inputs=+-|  SaturateOnIntegerOverflow=on  InputSameDT=on  OutDataTypeStr=Inherit: Same as first input
  Sum3 : Sum  Inputs=|++  SaturateOnIntegerOverflow=on  InputSameDT=on  OutDataTypeStr=Inherit: Same as first input
  Transposed rotation  matrix in yaw1 : marine_gnc/Models/ Kinematics/Transposed rotation  matrix in yaw  SystemSampleTime=-1
  "[-inf inf] to [-pi pi]" : marine_gnc/Utilities/Math Operations/[-inf inf] to [-pi pi]  SystemSampleTime=-1
  "[-inf inf] to [-pi pi]1" : marine_gnc/Utilities/Math Operations/[-inf inf] to [-pi pi]  SystemSampleTime=-1
  yaw angle : Fcn  Expr=u(3)
  tau : Outport  InitialOutput=0
  wires:
  Mux/1 -> Transposed rotation  matrix in yaw1/2
  Demux/1 -> Mux/1
  Demux/2 -> Mux/2
  eta_ref/1 -> Sum2/1
  Sum1/1 -> tau/1
  eta/1 -> yaw angle/1, Sum2/2
  Integrator/1 -> Ki/1
  Sum3/1 -> Sum1/1
  Transposed rotation  matrix in yaw1/1 -> Kp/1, Integrator/1
  Sum2/1 -> Demux/1  "regulation error"
  nu/1 -> Kd/1
  Kd/1 -> Demux3/1
  Reset_DP_integrator/1 -> Integrator/2
  yaw angle/1 -> "[-inf inf] to [-pi pi]1"/1  "psi"
  "[-inf inf] to [-pi pi]1"/1 -> Transposed rotation  matrix in yaw1/1
  Demux/3 -> "[-inf inf] to [-pi pi]"/1
  "[-inf inf] to [-pi pi]"/1 -> Mux/3
  Mux2/1 -> Sum1/2
  Demux1/1 -> K_p_surge_scale/1
  Demux1/2 -> K_p_sway_scale/1
  Demux1/3 -> K_p_yaw_scale/1
  K_p_surge_scale/1 -> Mux3/1
  K_p_yaw_scale/1 -> Mux3/3
  K_p_sway_scale/1 -> Mux3/2
  Kp/1 -> Demux1/1
  Mux3/1 -> Sum3/1
  Demux2/1 -> K_i_surge_scale/1
  Demux2/2 -> K_i_sway_scale/1
  Demux2/3 -> K_i_yaw_scale/1
  K_i_surge_scale/1 -> Mux1/1
  K_i_yaw_scale/1 -> Mux1/3
  K_i_sway_scale/1 -> Mux1/2
  Ki/1 -> Demux2/1
  Mux1/1 -> Sum3/2
  Demux3/1 -> K_d_surge_scale/1
  Demux3/2 -> K_d_sway_scale/1
  Demux3/3 -> K_d_yaw_scale/1
  K_d_surge_scale/1 -> Mux2/1
  K_d_yaw_scale/1 -> Mux2/3
  K_d_sway_scale/1 -> Mux2/2

== system DP/Control Systems/DP control/Thruster allocation ==
  tau : Inport
  f_act to u_act : Subsystem
  tau to f_act : Subsystem
  u_act : Outport
  wires:
  tau/1 -> tau to f_act/1(tau)
  tau to f_act/1(f_act) -> f_act to u_act/1(f_act)
  f_act to u_act/1(u_act) -> u_act/1

== system DP/Control Systems/PS3 u input control/Subsystem ==
  u_act : Inport  OutDataType=fixdt(1, 16)  OutScaling=2^0
  Bus Selector : BusSelector  OutputSignals=u_1,u_2,u_3,u_4,u_5
  Mux : Mux  Inputs=5
  f_act to tau : Subsystem
  u_act to f_act : Subsystem
  tau : Outport
  wires:
  u_act/1 -> Bus Selector/1
  f_act to tau/1(tau) -> tau/1
  u_act to f_act/1(f_act) -> f_act to tau/1(f_act)
  Mux/1 -> u_act to f_act/1(u_act)
  Bus Selector/1 -> Mux/1  "<u_1>"
  Bus Selector/2 -> Mux/2  "<u_2>"
  Bus Selector/3 -> Mux/3  "<u_3>"
  Bus Selector/4 -> Mux/4  "<u_4>"
  Bus Selector/5 -> Mux/5  "<u_5>"

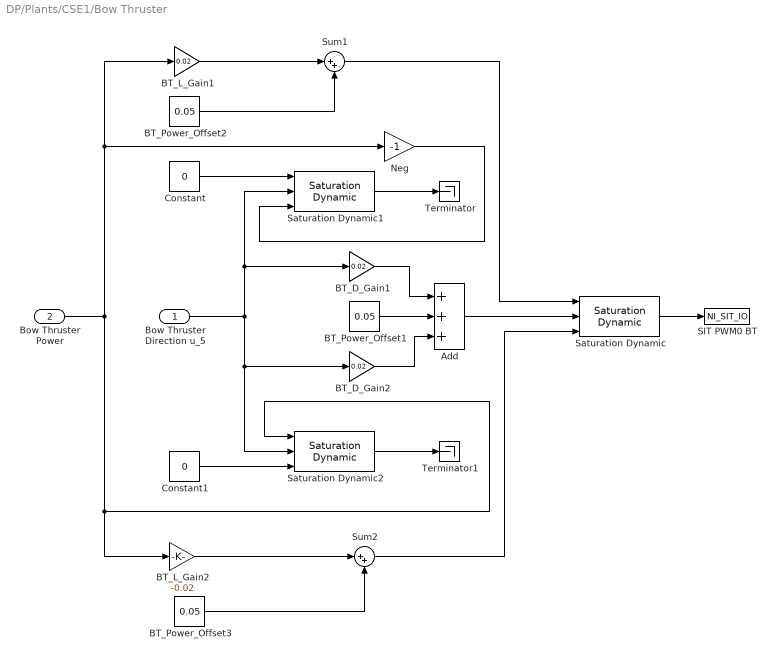
== system DP/Plants/CSE1/Bow Thruster ==
  Bow Thruster Direction u_5 : Inport
  Bow Thruster Power : Inport  Port=2
  Add : Sum  Inputs=+++
  BT_D_Gain1 : Gain  Gain=0.02
  BT_D_Gain2 : Gain  Gain=0.02
  BT_L_Gain1 : Gain  Gain=0.02
  BT_L_Gain2 : Gain  Gain=-0.02
  BT_Power_Offset1 : Constant  Value=0.05
  BT_Power_Offset2 : Constant  Value=0.05
  BT_Power_Offset3 : Constant  Value=0.05
  Constant : Constant  Value=0  OutDataType=fixdt(1, 16)  OutScaling=2^0
  Constant1 : Constant  Value=0  OutDataType=fixdt(1, 16)  OutScaling=2^0
  Neg : Gain  Gain=-1  ParameterDataType=fixdt(1, 16)  ParameterScaling=2^0  OutDataType=fixdt(1, 16)  OutScaling=2^0
  SIT PWM0 BT : S-Function  Priority=1  FunctionName=NI_SIT_IO  Parameters=width dtype portnum stime stype btype  EnableBusSupport=off  mask(SIT Outport){portnum=1, width=-1, stime=-1, dtype=auto, stype=auto, btype=0}
      mask prompts: portnum "Port number:"; width "Port dimensions (-1 for dynamically sized):"; stime "Sample time (-1 for inherited):"; dtype "Data type:"; stype "Signal type:"; btype "Block type:"
      mask help: Use this outport on any level of nested subsystems to allow the LabVIEW Simulation Interface Toolkit to map hardware to it.
      mask init:
      | NI_SIT_IO_init;
      settings: CopyFcn=NI_SIT_IO_callbacks(1);  DeleteFcn=NI_SIT_IO_callbacks(2);
      mask StyleString: edit,edit,edit,popup(auto|double|single|int8|uint8|int16|uint16|int32|uint32|boolean),popup(auto|real|complex),edit
      mask CallbackString: NI_SIT_IO_callbacks(3);|||NI_SIT_IO_callbacks(4);||
      mask TabNameString: Parameters,Parameters,Parameters,Parameters,Parameters,Parameters
      mask Display:
      | patch([-x x], [-y y], [.90980 .81960 .32156]);
      | plot([0 -x x 0], [rad -y y rad]);
      | fprintf('SIT%d', portnum);
  Saturation Dynamic : simulink/Discontinuities/Saturation Dynamic  SystemSampleTime=-1  OutMin=[]  OutMax=[]  OutDataTypeStr=Inherit: Same as second input  OutDataType=fixdt(1, 16)  OutScaling=2^-10  DoSatur=off
  Saturation Dynamic1 : simulink/Discontinuities/Saturation Dynamic  SystemSampleTime=-1  OutMin=[]  OutMax=[]  OutDataTypeStr=Inherit: Same as second input  OutDataType=fixdt(1, 16)  OutScaling=2^-10  DoSatur=off
  Saturation Dynamic2 : simulink/Discontinuities/Saturation Dynamic  SystemSampleTime=-1  OutMin=[]  OutMax=[]  OutDataTypeStr=Inherit: Same as second input  OutDataType=fixdt(1, 16)  OutScaling=2^-10  DoSatur=off
  Sum1 : Sum  Inputs=|++
  Sum2 : Sum  Inputs=|++
  Terminator : Terminator
  Terminator1 : Terminator
  wires:
  Bow Thruster Direction u_5/1 -> BT_D_Gain1/1, Saturation Dynamic1/2, BT_D_Gain2/1, Saturation Dynamic2/2
  BT_D_Gain1/1 -> Add/1
  BT_D_Gain2/1 -> Add/3
  BT_Power_Offset1/1 -> Add/2
  Add/1 -> Saturation Dynamic/2
  Bow Thruster Power/1 -> BT_L_Gain2/1, Saturation Dynamic2/1, BT_L_Gain1/1, Neg/1
  Sum1/1 -> Saturation Dynamic/1
  BT_L_Gain1/1 -> Sum1/1
  BT_L_Gain2/1 -> Sum2/1
  Sum2/1 -> Saturation Dynamic/3
  BT_Power_Offset2/1 -> Sum1/2
  BT_Power_Offset3/1 -> Sum2/2
  Saturation Dynamic/1 -> SIT PWM0 BT/1
  Saturation Dynamic2/1 -> Terminator1/1
  Saturation Dynamic1/1 -> Terminator/1
  Constant/1 -> Saturation Dynamic1/1
  Constant1/1 -> Saturation Dynamic2/3
  Neg/1 -> Saturation Dynamic1/3

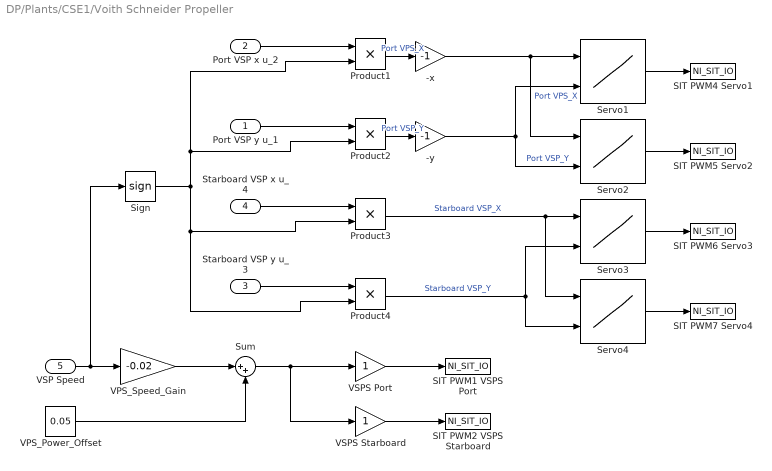
== system DP/Plants/CSE1/Voith Schneider Propeller  ==
  Port VSP y u_1 : Inport
  Port VSP x u_2 : Inport  Port=2
  Starboard VSP y u_3 : Inport  Port=3
  Starboard VSP x u_4 : Inport  Port=4
  VSP Speed : Inport  Port=5
  -x : Gain  Gain=-1
  -y : Gain  Gain=-1
  Product{1..4} (4 alike) : Product  RndMeth=Zero
  SIT PWM1 VSPS Port : S-Function  Priority=5  FunctionName=NI_SIT_IO  Parameters=width dtype portnum stime stype btype  EnableBusSupport=off  mask(SIT Outport){portnum=5, width=-1, stime=-1, dtype=auto, stype=auto, btype=0}
      mask prompts: portnum "Port number:"; width "Port dimensions (-1 for dynamically sized):"; stime "Sample time (-1 for inherited):"; dtype "Data type:"; stype "Signal type:"; btype "Block type:"
      mask help: Use this outport on any level of nested subsystems to allow the LabVIEW Simulation Interface Toolkit to map hardware to it.
      mask init:
      | NI_SIT_IO_init;
      settings: CopyFcn=NI_SIT_IO_callbacks(1);  DeleteFcn=NI_SIT_IO_callbacks(2);
      mask StyleString: edit,edit,edit,popup(auto|double|single|int8|uint8|int16|uint16|int32|uint32|boolean),popup(auto|real|complex),edit
      mask CallbackString: NI_SIT_IO_callbacks(3);|||NI_SIT_IO_callbacks(4);||
      mask TabNameString: Parameters,Parameters,Parameters,Parameters,Parameters,Parameters
      mask Display:
      | patch([-x x], [-y y], [.90980 .81960 .32156]);
      | plot([0 -x x 0], [rad -y y rad]);
      | fprintf('SIT%d', portnum);
  SIT PWM2 VSPS Starboard : S-Function  Priority=6  FunctionName=NI_SIT_IO  Parameters=width dtype portnum stime stype btype  EnableBusSupport=off  mask(SIT Outport){portnum=6, width=-1, stime=-1, dtype=auto, stype=auto, btype=0}
      mask prompts: portnum "Port number:"; width "Port dimensions (-1 for dynamically sized):"; stime "Sample time (-1 for inherited):"; dtype "Data type:"; stype "Signal type:"; btype "Block type:"
      mask help: Use this outport on any level of nested subsystems to allow the LabVIEW Simulation Interface Toolkit to map hardware to it.
      mask init:
      | NI_SIT_IO_init;
      settings: CopyFcn=NI_SIT_IO_callbacks(1);  DeleteFcn=NI_SIT_IO_callbacks(2);
      mask StyleString: edit,edit,edit,popup(auto|double|single|int8|uint8|int16|uint16|int32|uint32|boolean),popup(auto|real|complex),edit
      mask CallbackString: NI_SIT_IO_callbacks(3);|||NI_SIT_IO_callbacks(4);||
      mask TabNameString: Parameters,Parameters,Parameters,Parameters,Parameters,Parameters
      mask Display:
      | patch([-x x], [-y y], [.90980 .81960 .32156]);
      | plot([0 -x x 0], [rad -y y rad]);
      | fprintf('SIT%d', portnum);
  SIT PWM4 Servo1 : S-Function  Priority=1  FunctionName=NI_SIT_IO  Parameters=width dtype portnum stime stype btype  EnableBusSupport=off  mask(SIT Outport){portnum=1, width=-1, stime=-1, dtype=auto, stype=auto, btype=0}
      mask prompts: portnum "Port number:"; width "Port dimensions (-1 for dynamically sized):"; stime "Sample time (-1 for inherited):"; dtype "Data type:"; stype "Signal type:"; btype "Block type:"
      mask help: Use this outport on any level of nested subsystems to allow the LabVIEW Simulation Interface Toolkit to map hardware to it.
      mask init:
      | NI_SIT_IO_init;
      settings: CopyFcn=NI_SIT_IO_callbacks(1);  DeleteFcn=NI_SIT_IO_callbacks(2);
      mask StyleString: edit,edit,edit,popup(auto|double|single|int8|uint8|int16|uint16|int32|uint32|boolean),popup(auto|real|complex),edit
      mask CallbackString: NI_SIT_IO_callbacks(3);|||NI_SIT_IO_callbacks(4);||
      mask TabNameString: Parameters,Parameters,Parameters,Parameters,Parameters,Parameters
      mask Display:
      | patch([-x x], [-y y], [.90980 .81960 .32156]);
      | plot([0 -x x 0], [rad -y y rad]);
      | fprintf('SIT%d', portnum);
  SIT PWM5 Servo2 : S-Function  Priority=2  FunctionName=NI_SIT_IO  Parameters=width dtype portnum stime stype btype  EnableBusSupport=off  mask(SIT Outport){portnum=2, width=-1, stime=-1, dtype=auto, stype=auto, btype=0}
      mask prompts: portnum "Port number:"; width "Port dimensions (-1 for dynamically sized):"; stime "Sample time (-1 for inherited):"; dtype "Data type:"; stype "Signal type:"; btype "Block type:"
      mask help: Use this outport on any level of nested subsystems to allow the LabVIEW Simulation Interface Toolkit to map hardware to it.
      mask init:
      | NI_SIT_IO_init;
      settings: CopyFcn=NI_SIT_IO_callbacks(1);  DeleteFcn=NI_SIT_IO_callbacks(2);
      mask StyleString: edit,edit,edit,popup(auto|double|single|int8|uint8|int16|uint16|int32|uint32|boolean),popup(auto|real|complex),edit
      mask CallbackString: NI_SIT_IO_callbacks(3);|||NI_SIT_IO_callbacks(4);||
      mask TabNameString: Parameters,Parameters,Parameters,Parameters,Parameters,Parameters
      mask Display:
      | patch([-x x], [-y y], [.90980 .81960 .32156]);
      | plot([0 -x x 0], [rad -y y rad]);
      | fprintf('SIT%d', portnum);
  SIT PWM6 Servo3 : S-Function  Priority=3  FunctionName=NI_SIT_IO  Parameters=width dtype portnum stime stype btype  EnableBusSupport=off  mask(SIT Outport){portnum=3, width=-1, stime=-1, dtype=auto, stype=auto, btype=0}
      mask prompts: portnum "Port number:"; width "Port dimensions (-1 for dynamically sized):"; stime "Sample time (-1 for inherited):"; dtype "Data type:"; stype "Signal type:"; btype "Block type:"
      mask help: Use this outport on any level of nested subsystems to allow the LabVIEW Simulation Interface Toolkit to map hardware to it.
      mask init:
      | NI_SIT_IO_init;
      settings: CopyFcn=NI_SIT_IO_callbacks(1);  DeleteFcn=NI_SIT_IO_callbacks(2);
      mask StyleString: edit,edit,edit,popup(auto|double|single|int8|uint8|int16|uint16|int32|uint32|boolean),popup(auto|real|complex),edit
      mask CallbackString: NI_SIT_IO_callbacks(3);|||NI_SIT_IO_callbacks(4);||
      mask TabNameString: Parameters,Parameters,Parameters,Parameters,Parameters,Parameters
      mask Display:
      | patch([-x x], [-y y], [.90980 .81960 .32156]);
      | plot([0 -x x 0], [rad -y y rad]);
      | fprintf('SIT%d', portnum);
  SIT PWM7 Servo4 : S-Function  Priority=4  FunctionName=NI_SIT_IO  Parameters=width dtype portnum stime stype btype  EnableBusSupport=off  mask(SIT Outport){portnum=4, width=-1, stime=-1, dtype=auto, stype=auto, btype=0}
      mask prompts: portnum "Port number:"; width "Port dimensions (-1 for dynamically sized):"; stime "Sample time (-1 for inherited):"; dtype "Data type:"; stype "Signal type:"; btype "Block type:"
      mask help: Use this outport on any level of nested subsystems to allow the LabVIEW Simulation Interface Toolkit to map hardware to it.
      mask init:
      | NI_SIT_IO_init;
      settings: CopyFcn=NI_SIT_IO_callbacks(1);  DeleteFcn=NI_SIT_IO_callbacks(2);
      mask StyleString: edit,edit,edit,popup(auto|double|single|int8|uint8|int16|uint16|int32|uint32|boolean),popup(auto|real|complex),edit
      mask CallbackString: NI_SIT_IO_callbacks(3);|||NI_SIT_IO_callbacks(4);||
      mask TabNameString: Parameters,Parameters,Parameters,Parameters,Parameters,Parameters
      mask Display:
      | patch([-x x], [-y y], [.90980 .81960 .32156]);
      | plot([0 -x x 0], [rad -y y rad]);
      | fprintf('SIT%d', portnum);
  Servo1 : Lookup2D  RowIndex=[-1,0,1]  ColumnIndex=[-1,0,1]  Table=reshape([0.06,0.0495363,0.043301,0.06,0.052446,0.043301,0.06,0.0541518,0.043301],3,3)
  Servo2 : Lookup2D  RowIndex=[-1,0,1]  ColumnIndex=[-1,0,1]  Table=reshape([0.03860880,0.0386088,0.03860880,0.0459941,0.0477243,0.0500953,0.057,0.057,0.057],3,3)
  Servo3 : Lookup2D  RowIndex=[-1,0,1]  ColumnIndex=[-1,0,1]  Table=reshape([0.0640809,0.0640809,0.0640809,0.0539629,0.0541315,0.0556492,0.0442664,0.0442664,0.0442664],3,3)
  Servo4 : Lookup2D  RowIndex=[-1,0,1]  ColumnIndex=[-1,0,1]  Table=reshape([0.0602867,0.0470489,0.0403879,0.0602867,0.049747,0.0403879,0.0602867,0.0526138,0.0403879],3,3)
  Sign : Signum
  Sum : Sum  Inputs=|++
  VPS_Power_Offset : Constant  Value=0.05
  VPS_Speed_Gain : Gain  Gain=-0.02
  VSPS Port : Gain  ParameterDataType=fixdt(1, 16)  ParameterScaling=2^0  OutDataType=fixdt(1, 16)  OutScaling=2^0
  VSPS Starboard : Gain  ParameterDataType=fixdt(1, 16)  ParameterScaling=2^0  OutDataType=fixdt(1, 16)  OutScaling=2^0
  wires:
  Sign/1 -> Product1/2, Product2/2, Product3/2, Product4/2
  Product1/1 -> -x/1  "Port VPS_X"
  Product2/1 -> -y/1  "Port VSP_Y"
  Servo1/1 -> SIT PWM4 Servo1/1
  Servo2/1 -> SIT PWM5 Servo2/1
  Product3/1 -> Servo3/1, Servo4/1  "Starboard VSP_X"
  Product4/1 -> Servo3/2, Servo4/2  "Starboard VSP_Y"
  Servo3/1 -> SIT PWM6 Servo3/1
  Servo4/1 -> SIT PWM7 Servo4/1
  VSP Speed/1 -> VPS_Speed_Gain/1, Sign/1
  VPS_Speed_Gain/1 -> Sum/1
  VPS_Power_Offset/1 -> Sum/2
  Sum/1 -> VSPS Port/1, VSPS Starboard/1
  -y/1 -> Servo2/2, Servo1/2  "Port VSP_Y"
  -x/1 -> Servo1/1, Servo2/1  "Port VPS_X"
  Starboard VSP y u_3/1 -> Product4/1
  Starboard VSP x u_4/1 -> Product3/1
  Port VSP y u_1/1 -> Product2/1
  Port VSP x u_2/1 -> Product1/1
  VSPS Port/1 -> SIT PWM1 VSPS Port/1
  VSPS Starboard/1 -> SIT PWM2 VSPS Starboard/1

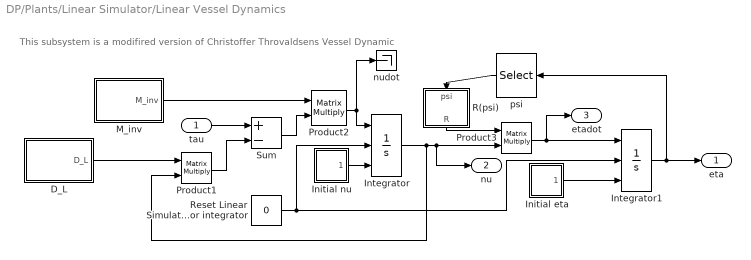
== system DP/Plants/Linear Simulator/Linear Vessel Dynamics ==
  note: This subsystem is a modifired version of Christoffer Throvaldsens Vessel Dynamic
  tau : Inport
  D_L : Subsystem
  Initial eta : Subsystem
  Initial nu : Subsystem
  Integrator : Integrator  ExternalReset=level  InitialConditionSource=external  InitialCondition=v1_0_real  UpperSaturationLimit=velocitySatValues1  LowerSaturationLimit=-1*velocitySatValues1
  Integrator1 : Integrator  ExternalReset=level  InitialConditionSource=external  InitialCondition=eta1_0_real
  M_inv : Subsystem
  Product1 : Product  Multiplication=Matrix(*)  RndMeth=Zero
  Product2 : Product  Multiplication=Matrix(*)  RndMeth=Zero
  Product3 : Product  Multiplication=Matrix(*)  RndMeth=Zero
  R(psi) : Subsystem
  Reset Linear Simulator integrator : Constant  Value=0
  Sum : Sum  Inputs=+-
  nudot : Terminator
  psi : Selector  InputPortWidth=3  IndexOptions=Index vector (dialog)  Indices=[3]  OutputSizes=1
  eta : Outport
  nu : Outport  Port=2
  etadot : Outport  Port=3
  wires:
  Sum/1 -> Product2/2
  Product2/1 -> Integrator/1, nudot/1
  Integrator/1 -> Product1/2, nu/1, Product3/2
  R(psi)/1(R) -> Product3/1
  psi/1 -> R(psi)/1(psi)
  M_inv/1(M_inv) -> Product2/1
  tau/1 -> Sum/1
  Product1/1 -> Sum/2
  Product3/1 -> etadot/1, Integrator1/1
  Integrator1/1 -> psi/1, eta/1
  Initial nu/1(nu_0) -> Integrator/3
  Reset Linear Simulator integrator/1 -> Integrator/2, Integrator1/2
  Initial eta/1(eta_0) -> Integrator1/3
  D_L/1(D_L) -> Product1/1

== system DP/Control Systems/DP control/Thruster allocation/f_act to u_act ==
  f_act : Inport
  Demux : Demux  Outputs=5
  Mux : Mux  Inputs=5
  f_1 to u_1 : Subsystem
  f_2 to u_2 : Subsystem
  f_3 to u_3 : Subsystem
  f_4 to u_4 : Subsystem
  f_5 to u_5 : Subsystem
  u_act : Outport
  wires:
  f_5 to u_5/1(u_5) -> Mux/5
  f_4 to u_4/1(u_4) -> Mux/4
  f_3 to u_3/1(u_3) -> Mux/3
  f_2 to u_2/1(u_2) -> Mux/2
  f_1 to u_1/1(u_1) -> Mux/1
  Demux/5 -> f_5 to u_5/1(f_5)
  Demux/4 -> f_4 to u_4/1(f_4)
  Demux/3 -> f_3 to u_3/1(f_3)
  Demux/1 -> f_1 to u_1/1(f_1)
  Mux/1 -> u_act/1
  f_act/1 -> Demux/1
  Demux/2 -> f_2 to u_2/1(f_2)

== system DP/Control Systems/DP control/Thruster allocation/tau to f_act ==
  tau : Inport
  Product : Product  Multiplication=Matrix(*)  OutDataType=fixdt(1, 16)  OutScaling=2^0  RndMeth=Zero
  Pseudoinverse : dspinverses/Pseudoinverse  wanterr=off
  T_e : Subsystem
  f_act : Outport
  wires:
  Product/1 -> f_act/1
  tau/1 -> Product/2
  Pseudoinverse/1 -> Product/1
  T_e/1(T_e) -> Pseudoinverse/1

== system DP/Control Systems/PS3 u input control/Subsystem/f_act to tau ==
  f_act : Inport
  Product : Product  Multiplication=Matrix(*)  OutDataType=fixdt(1, 16)  OutScaling=2^0  RndMeth=Zero
  T_e : Subsystem
  tau : Outport
  wires:
  f_act/1 -> Product/2
  T_e/1(T_e) -> Product/1
  Product/1 -> tau/1
